simulink model "SB4_bus_done"  (R2024b)
settings: Solver=FixedStepDiscrete  StartTime=0.0  StopTime=1  FixedStep=0.05  RelTol=1e-3
settings Model: Creator=admin  LastModifiedBy=admin

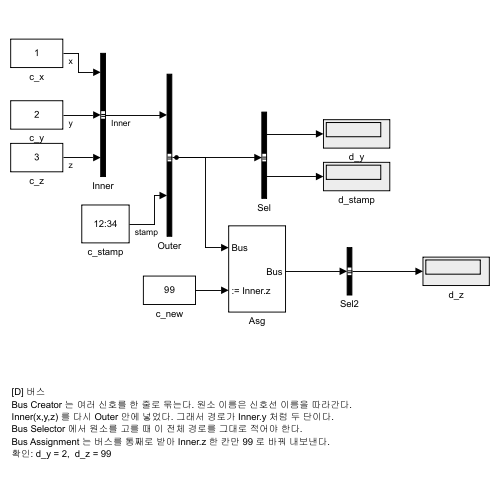
[thumbnail: Simulink's stored preview of the top-level diagram]
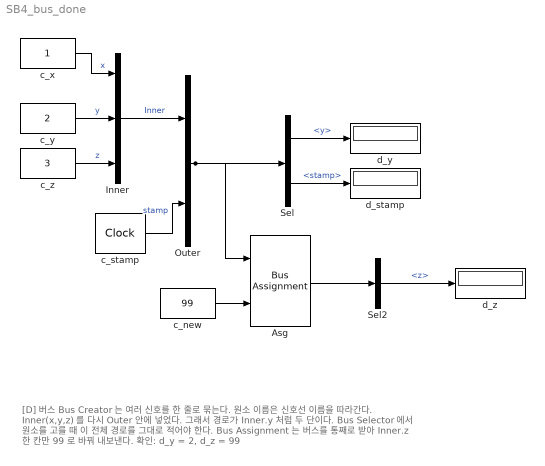
== system SB4_bus_done ==
  note: [D] 버스
      | Bus Creator 는 여러 신호를 한 줄로 묶는다. 원소 이름은 신호선 이름을 따라간다.
      | Inner(x,y,z) 를 다시 Outer 안에 넣었다. 그래서 경로가 Inner.y 처럼 두 단이다.
      | Bus Selector 에서 원소를 고를 때 이 전체 경로를 그대로 적어야 한다.
      | Bus Assignment 는 버스를 통째로 받아 Inner.z 한 칸만 99 로 바꿔 내보낸다.
      | 확인: d_y = 2,  d_z = 99
  Asg : BusAssignment  AssignedSignals=Inner.z
  Inner : BusCreator  Inputs=3
  Outer : BusCreator  Inputs=2
  Sel : BusSelector  OutputSignals=Inner.y,stamp
  Sel2 : BusSelector  OutputSignals=Inner.z
  c_new : Constant  Value=99
  c_stamp : DigitalClock  SampleTime=0.05
  c_x : Constant
  c_y : Constant  Value=2
  c_z : Constant  Value=3
  d_stamp : Display
  d_y : Display
  d_z : Display
  wires:
  Inner/1 -> Outer/1  "Inner"
  c_y/1 -> Inner/2  "y"
  c_x/1 -> Inner/1  "x"
  c_stamp/1 -> Outer/2  "stamp"
  c_z/1 -> Inner/3  "z"
  Sel/1 -> d_y/1  "<y>"
  Outer/1 -> Sel/1, Asg/1
  c_new/1 -> Asg/2
  Sel/2 -> d_stamp/1  "<stamp>"
  Asg/1 -> Sel2/1
  Sel2/1 -> d_z/1  "<z>"
